simulink model "main"  (R2022a)
settings: Solver=ode4  StartTime=0.0  StopTime=5730.76  FixedStep=0.1  RelTol=1e-3
undefined symbols (not defined in the file): X, Y, Z
libraries: nesl_utility x25, sm_lib x9, sharedtransform x4, aerolibutil x2, sharedutil x1
(part 2 of 2)

== matlab function main/Ephemerides Date1/Modified Julian Date (mjd0) ==
  data: dmy input; diju output
function diju  =  djm (dmy)
% [diju] = djm (day, month, year)
%    The function djm furnishes the Modified Julian
%    Date with reference to the day, month and year,
%    at zero hours of the day.
% inputs:
%   dmy(1): day, day of the month
%   dmy(2): month, month of the year
%   dmy(3): year

% outputs:
%   diju
%       Modified Julian Date in days, referred to 1950.0. 
%
% Valdemir Carrara, Apr, 2003
%

diju = 367*dmy(3) + dmy(1) - 712269 + fix(275*dmy(2)/9)- fix(7*(dmy(3)+fix((dmy(2)+9)/12))/4);
